simulink model "prueba5"  (R2022a)
settings: Solver=VariableStepAuto  StartTime=0.0  StopTime=60  RelTol=1e-3
values from neighbouring files (symbols this model uses):
  A = A(4:10,4:10)    [linealControl.m]    (also in linealYcontrol5.m)
  B = B(4:10,:)    [linealControl.m]    (also in linealYcontrol5.m)
  int5 = [0.0001,0.0001,0.0001,0.0001,0.0001,0.0001,0.0001,0.0001,0.0001,0.0001]    [linealControl.m]    (also in linealYcontrol5.m)
  KA = ak1    [linealControl.m]    (also in linealYcontrol5.m)
  KB = bk1    [linealControl.m]    (also in linealYcontrol5.m)
  KC = ck1    [linealControl.m]    (also in linealYcontrol5.m)
  KD = dk1    [linealControl.m]    (also in linealYcontrol5.m)
undefined symbols (not defined in the file or in its folder): lineal5simu
settings Model: Creator=LENOVO  LastModifiedBy=LENOVO
settings DebuggingCC: UnconnectedInputMsg=warning  UnconnectedOutputMsg=warning  UnconnectedLineMsg=warning
settings RTWCC: DLArmComputeVersion=19.05

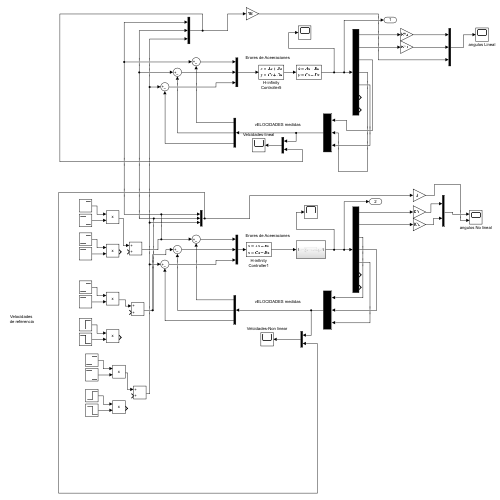
[thumbnail: Simulink's stored preview of the top-level diagram]
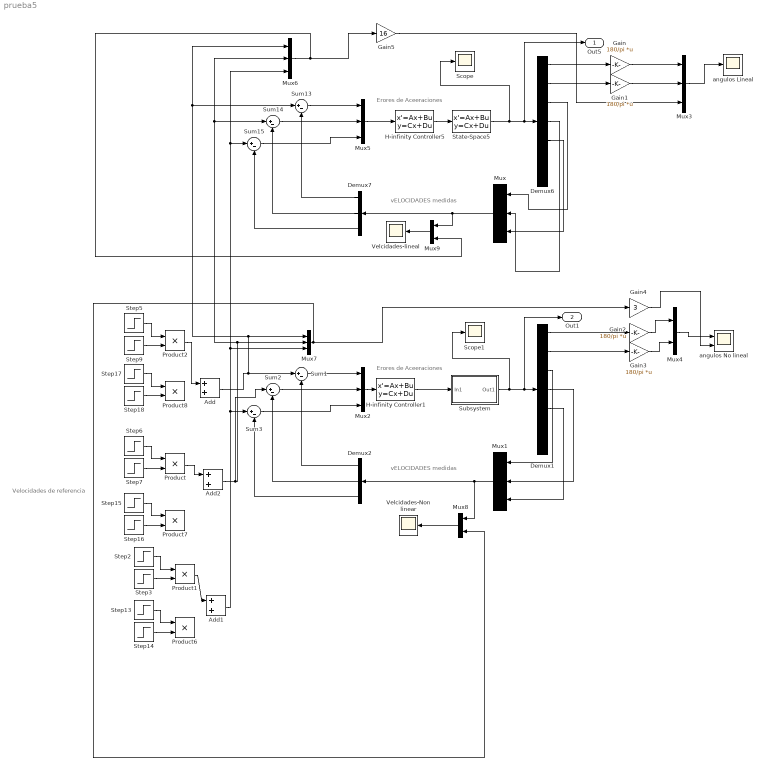
== system prueba5 ==
  note: Erores de Aceeraciones
  note: vELOCIDADES medidas
  note: vELOCIDADES medidas
  note: Erores de Aceeraciones
  note: Velocidades
      | de referencia
  Add : Sum
  Add1 : Sum
  Add2 : Sum
  Demux1 : Demux  Outputs=7
  Demux2 : Demux  Outputs=3
  Demux6 : Demux  Outputs=7
  Demux7 : Demux  Outputs=3
  Gain{,1..3} (4 alike) : Gain  Gain=180/pi  Multiplication=Matrix(K*u)
  Gain4 : Gain  Gain=3
  Gain5 : Gain  Gain=16
  H-infinity Controller1 : StateSpace  A=KA  B=KB  C=KC  D=KD  InitialCondition=0
  H-infinity Controller5 : StateSpace  A=KA  B=KB  C=KC  D=KD  InitialCondition=0
  Mux{,1..3,5..7} (7 alike) : Mux  Inputs=3
  Mux4 : Mux  Inputs=2
  Mux8 : Mux  Inputs=2
  Mux9 : Mux  Inputs=2
  Product{,1..2,6..8} (6 alike) : Product
  Scope : Scope
  Scope1 : Scope
  State-Space5 : StateSpace  A=A  B=B  C=eye(7)  D=zeros(7,3)  InitialCondition=0  ParameterTunability=Unconstrained
  Step13 : Step  Time=50  After=5  SampleTime=0
  Step14 : Step  Time=65  Before=1  After=0  SampleTime=0
  Step15 : Step  Time=60  After=5  SampleTime=0
  Step16 : Step  Time=75  Before=1  After=0  SampleTime=0
  Step17 : Step  Time=240  After=10  SampleTime=0
  Step18 : Step  Time=70  Before=1  After=0  SampleTime=0
  Step2 : Step  Time=15  After=5  SampleTime=0
  Step3 : Step  Time=30  Before=1  After=0  SampleTime=0
  Step5 : Step  Time=20  After=5  SampleTime=0
  Step6 : Step  Time=25  After=5  SampleTime=0
  Step7 : Step  Time=40  Before=1  After=0  SampleTime=0
  Step9 : Step  Time=35  Before=1  After=0  SampleTime=0
  Subsystem : Subsystem
  Sum{1..3,13..15} (6 alike) : Sum  Inputs=|+-
  Velcidades-Non linear : Scope
  Velcidades-lineal : Scope
  angulos Lineal : Scope
  angulos No lineal : Scope  NumInputPorts=2
  Out5 : Outport
  Out1 : Outport  Port=2
  wires:
  H-infinity Controller5/1 -> State-Space5/1
  Sum14/1 -> Mux5/2
  State-Space5/1 -> Scope/1, Out5/1, Demux6/1
  Demux7/1 -> Sum13/2
  Sum13/1 -> Mux5/1
  Mux5/1 -> H-infinity Controller5/1
  Demux7/3 -> Sum15/2
  Sum15/1 -> Mux5/3
  Mux/1 -> Mux9/1, Demux7/1
  Demux7/2 -> Sum14/2
  Sum3/1 -> Mux2/3
  Demux2/1 -> Sum1/2
  Mux1/1 -> Mux8/1, Demux2/1
  Sum1/1 -> Mux2/1
  Demux2/2 -> Sum2/2
  Demux2/3 -> Sum3/2
  Sum2/1 -> Mux2/2
  Subsystem/1(Out1) -> Scope1/1, Out1/1, Demux1/1
  Gain1/1 -> Mux3/2
  Mux3/1 -> angulos Lineal/1
  Gain/1 -> Mux3/1
  Mux4/1 -> angulos No lineal/1
  Gain3/1 -> Mux4/2
  Gain2/1 -> Mux4/1
  Mux2/1 -> H-infinity Controller1/1
  H-infinity Controller1/1 -> Subsystem/1(In1)
  Demux6/1 -> Gain/1
  Demux6/2 -> Gain1/1
  Demux6/3 -> Mux/1
  Demux6/4 -> Mux/2
  Demux6/5 -> Mux/3
  Demux1/1 -> Gain2/1
  Demux1/2 -> Gain3/1
  Demux1/3 -> Mux1/1
  Demux1/4 -> Mux1/2
  Demux1/5 -> Mux1/3
  Mux7/1 -> Gain4/1, Mux8/2
  Mux6/1 -> Gain5/1, Mux9/2
  Gain5/1 -> Mux3/3
  Mux9/1 -> Velcidades-lineal/1
  Mux8/1 -> Velcidades-Non linear/1
  Step6/1 -> Product/1
  Step7/1 -> Product/2
  Step2/1 -> Product1/1
  Step3/1 -> Product1/2
  Step5/1 -> Product2/1
  Step9/1 -> Product2/2
  Product2/1 -> Add/1
  Product1/1 -> Add1/1
  Product/1 -> Add2/1
  Add/1 -> Mux7/1, Sum13/1, Mux6/1, Sum1/1
  Add1/1 -> Sum15/1, Mux6/3, Mux7/3, Sum3/1
  Step13/1 -> Product6/1
  Step14/1 -> Product6/2
  Step15/1 -> Product7/1
  Step16/1 -> Product7/2
  Step17/1 -> Product8/1
  Step18/1 -> Product8/2
  Add2/1 -> Sum14/1, Mux6/2, Mux7/2, Sum2/1
  Gain4/1 -> angulos No lineal/2

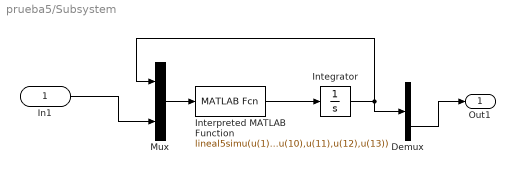
== system prueba5/Subsystem ==
  In1 : Inport
  Demux : Demux  Outputs=[3 7]
  Integrator : Integrator  InitialCondition=int5
  Interpreted MATLAB Function : MATLABFcn  MATLABFcn=lineal5simu(u(1),u(2),u(3),u(4),u(5),u(6),u(7),u(8),u(9),u(10),u(11),u(12),u(13))
  Mux : Mux  Inputs=[10 3]
  Out1 : Outport
  wires:
  Interpreted MATLAB Function/1 -> Integrator/1
  Integrator/1 -> Demux/1, Mux/1
  Mux/1 -> Interpreted MATLAB Function/1
  In1/1 -> Mux/2
  Demux/2 -> Out1/1
